simulink model "Fault_Analyzer_Example_FaultModel_2"  (R2025b)
settings: Solver=VariableStepAuto  StartTime=0.0  StopTime=10.0  RelTol=1e-3  EnableMultiTasking=on
settings Model: Creator=georg  LastModifiedBy=georg
settings DebuggingCC: InheritedTsInSrcMsg=none

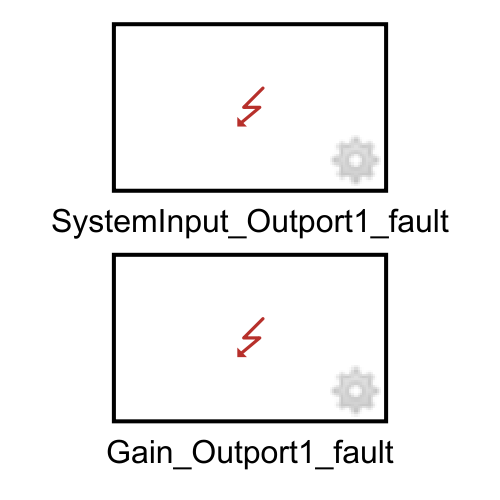
[thumbnail: Simulink's stored preview of the top-level diagram]
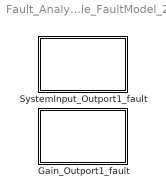
== system Fault_Analyzer_Example_FaultModel_2 ==
  Gain_Outport1_fault : Subsystem  TreatAsAtomicUnit=on  IsInjectorSS=on
  SystemInput_Outport1_fault : Subsystem  TreatAsAtomicUnit=on  IsInjectorSS=on

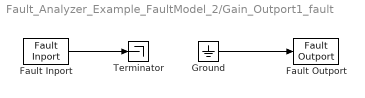
== system Fault_Analyzer_Example_FaultModel_2/Gain_Outport1_fault ==
  Fault Inport : FaultInport
  Fault Outport : FaultOutport
  Ground : Ground
  Terminator : Terminator
  wires:
  Ground/1 -> Fault Outport/1
  Fault Inport/1 -> Terminator/1

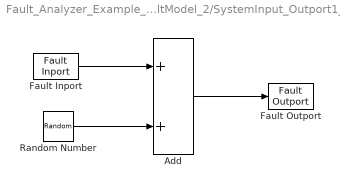
== system Fault_Analyzer_Example_FaultModel_2/SystemInput_Outport1_fault ==
  Add : Sum
  Fault Inport : FaultInport
  Fault Outport : FaultOutport
  Random Number : RandomNumber  SampleTime=0.1
  wires:
  Fault Inport/1 -> Add/1
  Random Number/1 -> Add/2
  Add/1 -> Fault Outport/1
